simulink model "Adelanto_digital_EsquemaSimulink"  (R2020a)
settings: Solver=ode45  StartTime=0.0  StopTime=10  MaxStep=1e-5  RelTol=1e-3  EnableMultiTasking=on
undefined symbols (not defined in the file): cc, k, p1, p2, pc, Tm
settings Model: Creator=Usuario  LastModifiedBy=mauri
settings DataIOCC: SaveFormat=Array  SignalLoggingSaveFormat=ModelDataLogs  ReturnWorkspaceOutputs=off
settings OptimizationCC: InitFltsAndDblsToZero=on  LifeSpan=inf
settings DebuggingCC: SaveWithParameterizedLinksMsg=none  UnderspecifiedInitializationDetection=Classic  MergeDetectMultiDrivingBlocksExec=none  SignalResolutionControl=TryResolveAllWithWarning  SolverPrmCheckMsg=warning  MultiTaskDSMMsg=warning  MultiTaskCondExecSysMsg=none  FcnCallInpInsideContextMsg=warning  SFUnexpectedBacktrackingDiag=warning  SFNoUnconditionalDefaultTransitionDiag=warning  SFExecutionAtInitializationDiag=none  ArithmeticOperatorsInVariantConditions=warning
settings HardwareCC: ProdBitPerPointer=32  ProdBitPerSizeT=32  ProdBitPerPtrDiffT=32  ProdLargestAtomicFloat=None  ProdIntDivRoundTo=Undefined  ProdEndianess=Unspecified  ProdWordSize=32  ProdHWDeviceType=32-bit Generic
settings ModelReferenceCC: PropagateSignalLabelsOutOfModel=off
settings SFSimCC: SimUseLocalCustomCode=off  CustomCodeUndefinedFunction=UseInterfaceOnly
settings RTWCC: RTWUseLocalCustomCode=off
settings CodeAppCC: StateflowObjectComments=on
settings GRTTargetCC: TargetFcnLib=ansi_tfl_tmw.mat  TargetLangStandard=C89/C90 (ANSI)  CombineOutputUpdateFcns=off  GRTInterface=on
settings ConfigComp: CovMetricSettings=dw  CovHtmlReporting=on  CovSaveCumulativeToWorkspaceVar=on  CovSaveSingleToWorkspaceVar=on  CovExternalEMLEnable=off  CovSFcnEnable=off

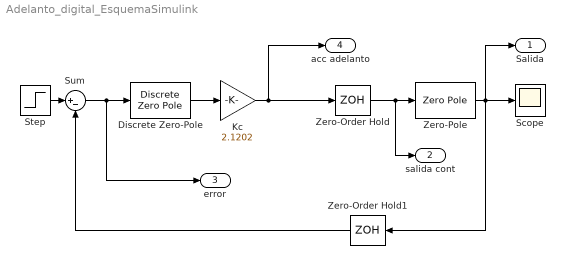
== system Adelanto_digital_EsquemaSimulink ==
  Discrete Zero-Pole : DiscreteZeroPole  Zeros=[cc]  Poles=[pc]  Gain=1  SampleTime=Tm
  Kc : Gain  Gain=2.1202
  Scope : Scope
  Step : Step  Time=0  SampleTime=Tm
  Sum : Sum  Inputs=|+-
  Zero-Order Hold : ZeroOrderHold  SampleTime=Tm
  Zero-Order Hold1 : ZeroOrderHold  SampleTime=Tm
  Zero-Pole : ZeroPole  Zeros=[]  Poles=[p1 p2]  Gain=k
  Salida : Outport
  salida cont : Outport  Port=2
  error : Outport  Port=3
  acc adelanto : Outport  Port=4
  wires:
  Zero-Order Hold/1 -> Zero-Pole/1, salida cont/1
  Step/1 -> Sum/1
  Zero-Pole/1 -> Zero-Order Hold1/1, Scope/1, Salida/1
  Zero-Order Hold1/1 -> Sum/2
  Sum/1 -> Discrete Zero-Pole/1, error/1
  Kc/1 -> Zero-Order Hold/1, acc adelanto/1
  Discrete Zero-Pole/1 -> Kc/1
